simulink model "variable_k_wrt_x"  (R2019b)
settings: Solver=ode45  StartTime=0.0  StopTime=50  RelTol=1e-4
libraries: simulink x1
settings Model: Creator=KEYUR  LastModifiedBy=KEYUR
settings DataIOCC: ExternalInput=[t, y]  LoadExternalInput=on

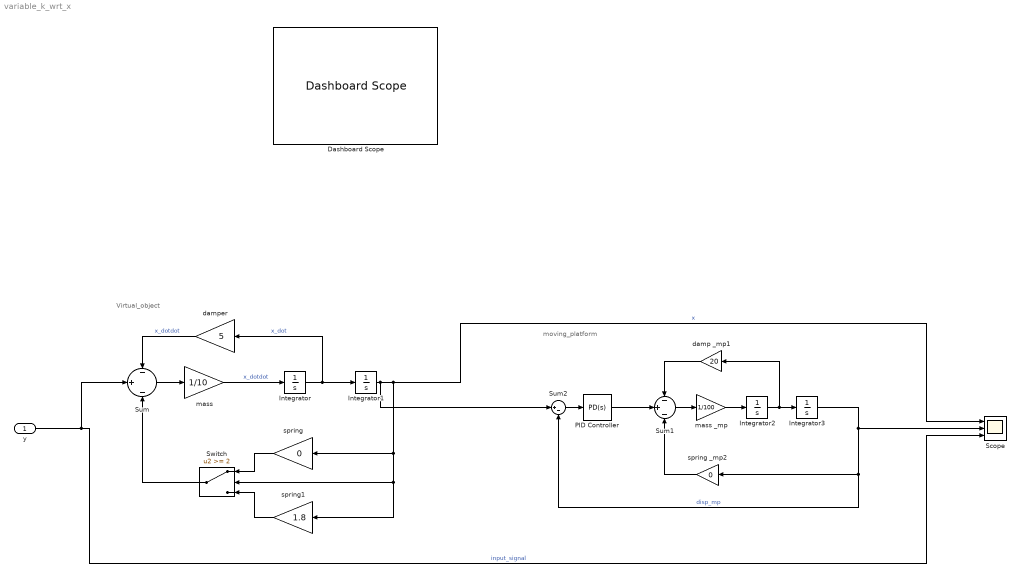
== system variable_k_wrt_x ==
  note: moving_platform
  note: Virtual_object
  y : Inport
  Dashboard Scope : DashboardScope
  Integrator{,1..3} (4 alike) : Integrator
  PID Controller : simulink/Continuous/PID Controller  Controller=PD  Form=Parallel  TimeDomain=Continuous-time  SampleTime=-1  IntegratorMethod=Forward Euler  FilterMethod=Forward Euler  ControllerParametersSource=internal  P=62.4207988719117  I=1  D=114.018935921912  UseFilter=on  N=141.149246616551  TunerSelectOption=Transfer Function Based (PID Tuner App)  InitialConditionSource=internal  InitialConditionForIntegrator=0  InitialConditionForFilter=0  DifferentiatorICPrevScaledInput=0  ExternalReset=none  TrackingMode=off  Kt=1  LimitOutput=off  UpperSaturationLimit=inf  LowerSaturationLimit=-inf  LinearizeAsGain=on  AntiWindupMode=none  Kb=1  POutMin=[]  POutMax=[]  IOutMin=[]  IOutMax=[]  DOutMin=[]  DOutMax=[]  NOutMin=[]  NOutMax=[]  SumOutMin=[]  SumOutMax=[]  SaturationOutMin=[]  SaturationOutMax=[]  PParamMin=[]  PParamMax=[]  IParamMin=[]  IParamMax=[]  DParamMin=[]  DParamMax=[]  NParamMin=[]  NParamMax=[]  KbParamMin=[]  KbParamMax=[]  KtParamMin=[]  KtParamMax=[]  KbOutMin=[]  KbOutMax=[]  KtOutMin=[]  KtOutMax=[]  IntegratorOutMin=[]  IntegratorOutMax=[]  FilterOutMin=[]  FilterOutMax=[]  SumI1OutMin=[]  SumI1OutMax=[]  SumI2OutMin=[]  SumI2OutMax=[]  SumI3OutMin=[]  SumI3OutMax=[]  SumI4OutMin=[]  SumI4OutMax=[]  SumDOutMin=[]  SumDOutMax=[]  DifferentiatorOutMin=[]  DifferentiatorOutMax=[]  FilterDiffOutCoefMin=[]  FilterDiffOutCoefMax=[]  ReciprocalOutMin=[]  ReciprocalOutMax=[]  SumDenOutMin=[]  SumDenOutMax=[]  SumNumOutMin=[]  SumNumOutMax=[]  DivideOutMin=[]  DivideOutMax=[]  IntegratorContinuousStateAttributes=''  IntegratorStateMustResolveToSignalObject=off  IntegratorRTWStateStorageClass=Auto  FilterContinuousStateAttributes=''  FilterStateMustResolveToSignalObject=off  FilterRTWStateStorageClass=Auto  ParallelPVariant=InternalParameters  IdealPVariant=Disabled  IVariant=Disabled  DVariant=InternalParameters  IntegratorVariant=Disabled  SatVariant=Disabled  AWVariant=Disabled  PCopyVariant=Disabled  TRVariant=Disabled  FdbkBlocksVariant=Forward  IdealPFdbkVariant=Disabled  SatFdbkVariant=Disabled  DerivativeFilterVariant=ContFilter  NVariant=InternalParameters  NCopyVariant=Disabled  FilterICVariant=InternalICsFilter  IntegratorICVariant=Disabled  ExternalResetVariant=Disabled  TRSumVariant=Passthrough  SumFdbkVariant=Disabled  SumVariant=Sum_PD
  Scope : Scope  NumInputPorts=3
  Sum : Sum  Inputs=-|+|-
  Sum1 : Sum  Inputs=-|+|-
  Sum2 : Sum  Inputs=|+-
  Switch : Switch  Threshold=2
  damp _mp1 : Gain  Gain=20
  damper : Gain  Gain=5
  mass : Gain  Gain=1/10
  mass _mp : Gain  Gain=1/100
  spring : Gain  Gain=0
  spring _mp2 : Gain  Gain=0
  spring1 : Gain  Gain=1.8
  wires:
  y/1 -> Sum/2, Scope/3  "input_signal"
  Sum/1 -> mass/1
  damper/1 -> Sum/1  "x_dotdot"
  spring1/1 -> Switch/3
  Switch/1 -> Sum/3
  spring/1 -> Switch/1
  mass/1 -> Integrator/1  "x_dotdot"
  Integrator1/1 -> spring1/1, Switch/2, spring/1, Scope/1, Sum2/1  "x"
  Integrator/1 -> damper/1, Integrator1/1  "x_dot"
  Integrator2/1 -> damp _mp1/1, Integrator3/1
  damp _mp1/1 -> Sum1/1
  mass _mp/1 -> Integrator2/1
  Sum1/1 -> mass _mp/1
  Integrator3/1 -> Scope/2, Sum2/2, spring _mp2/1  "disp_mp"
  PID Controller/1 -> Sum1/2
  spring _mp2/1 -> Sum1/3
  Sum2/1 -> PID Controller/1
